simulink model "A1_manual"  (R2012b)
settings: Solver=ode45  StartTime=0.0  StopTime=500  RelTol=1e-3
PreLoadFcn:
  | Initialize
StopFcn:
  | A1_plot_and_save
undefined symbols (not defined in the file or in its folder): P, PlotTanks2
libraries: simulink x4
settings Model: Creator=tsladeche  LastModifiedBy=John
settings DataIOCC: SignalLoggingSaveFormat=ModelDataLogs
settings DebuggingCC: FcnCallInpInsideContextMsg=UseLocalSettings  StrictBusMsg=Warning
settings GRTTargetCC: CombineOutputUpdateFcns=off  GRTInterface=on

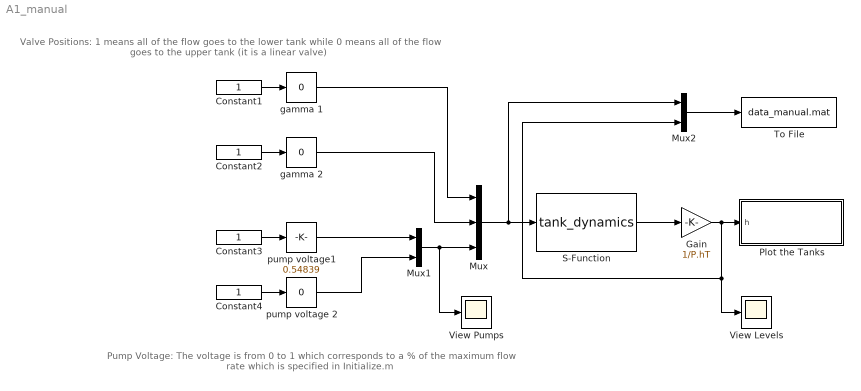
== system A1_manual ==
  note: Pump Voltage: The voltage is from 0 to 1 which corresponds
      | to a % of the maximum flow rate which is specified in Initialize.m
  note: Valve Positions: 1 means all of the flow goes to the lower tank
      | while 0 means all of the flow goes to the upper tank (it is a linear valve)
  Constant{1..4} (4 alike) : Constant
  Gain : Gain  Gain=1/P.hT
  Mux : Mux  Inputs=3
  Mux1 : Mux  Inputs=2
  Mux2 : Mux  Inputs=2
  Plot the Tanks : Subsystem
  S-Function : S-Function  FunctionName=tank_dynamics  Parameters=P  EnableBusSupport=off
  To File : ToFile  Filename=data_manual.mat  MatrixName=tanks  SampleTime=1
  View Levels : Scope
      settings: YMin=0  YMax=1
  View Pumps : Scope
  gamma 1 : simulink/Math Operations/Slider Gain  low=0  gain=0  high=1
  gamma 2 : simulink/Math Operations/Slider Gain  low=0  gain=0  high=1
  pump voltage 2 : simulink/Math Operations/Slider Gain  low=0  gain=0  high=1
  pump voltage1 : simulink/Math Operations/Slider Gain  low=0  gain=0.54839  high=1
  wires:
  Constant2/1 -> gamma 2/1
  Constant1/1 -> gamma 1/1
  gamma 1/1 -> Mux/1
  gamma 2/1 -> Mux/2
  Gain/1 -> Mux2/2, View Levels/1, Plot the Tanks/1(h)
  S-Function/1 -> Gain/1
  Constant3/1 -> pump voltage1/1
  Constant4/1 -> pump voltage 2/1
  Mux1/1 -> View Pumps/1, Mux/3
  pump voltage1/1 -> Mux1/1
  pump voltage 2/1 -> Mux1/2
  Mux/1 -> Mux2/1, S-Function/1
  Mux2/1 -> To File/1

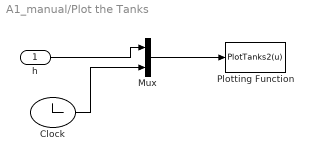
== system A1_manual/Plot the Tanks ==
  h : Inport
  Clock : Clock
  Mux : Mux  Inputs=2
  Plotting Function : MATLABFcn  MATLABFcn=PlotTanks2(u)  OutputDimensions=0  SampleTime=.05
  wires:
  Mux/1 -> Plotting Function/1
  Clock/1 -> Mux/2
  h/1 -> Mux/1
